simulink model "ModeleringBevegelserSim"  (R2023b)
settings: Solver=FixedStepAuto  StartTime=0.0  StopTime=6  FixedStep=1e-3  RelTol=1e-6
undefined symbols (not defined in the file): areal_front, areal_side, areal_topp, bidrag_gir_front, bidrag_gir_side, Cd_front, Cd_side, Cd_topp, g, masse, r_motor_gir, tetthet_vann, theta_motor_gir, treghetsmoment_gir
libraries: spsFirstOrderFilterLib x4, slpidlib x4
settings Model: Creator=bmm1  LastModifiedBy=bmm1

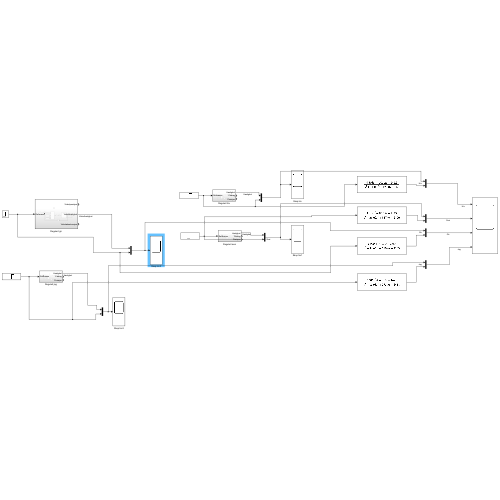
[thumbnail: Simulink's stored preview of the top-level diagram]
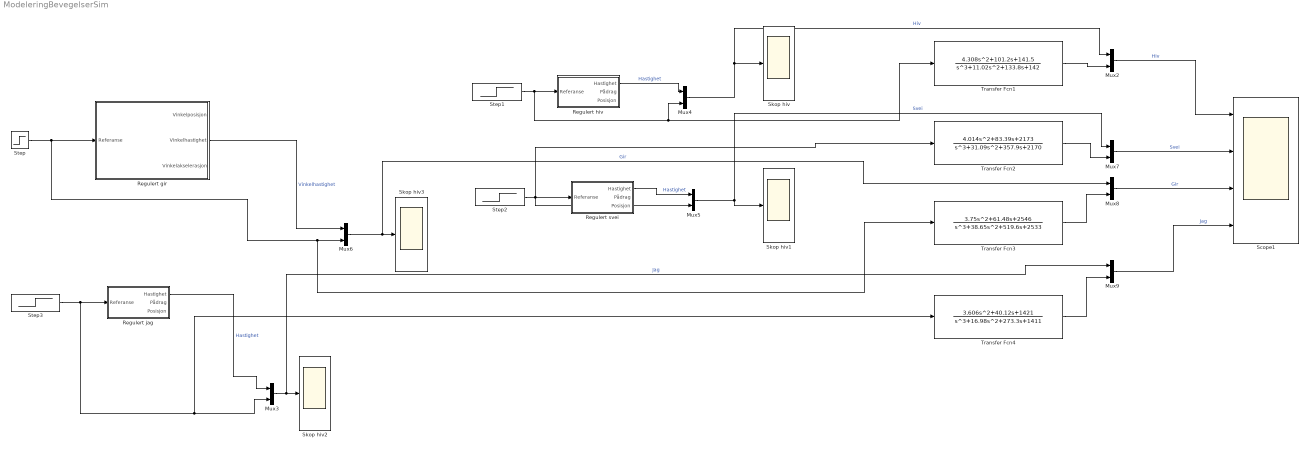
== system ModeleringBevegelserSim ==
  Mux{2..9} (8 alike) : Mux  Inputs=2
  "Regulert gir " : Subsystem
  Regulert hiv : Subsystem
  Regulert jag : Subsystem
  Regulert svei : Subsystem
  Scope1 : Scope  NumInputPorts=4
  Skop hiv{,1..3} (4 alike) : Scope
  Step : Step  SampleTime=0
  Step1 : Step  After=0.6  SampleTime=0
  Step2 : Step  After=0.4  SampleTime=0
  Step3 : Step  After=0.6  SampleTime=0
  Transfer Fcn1 : TransferFcn  Numerator=[4.308 101.2 141.5]  Denominator=[1 11.02 133.8 142]
  Transfer Fcn2 : TransferFcn  Numerator=[4.014 83.39 2173]  Denominator=[1 31.09 357.9 2170]
  Transfer Fcn3 : TransferFcn  Numerator=[3.75 61.48 2546]  Denominator=[1 38.65 519.6 2533]
  Transfer Fcn4 : TransferFcn  Numerator=[3.606 40.12 1421]  Denominator=[1 16.98 273.3 1411]
  wires:
  "Regulert gir "/2(Vinkelhastighet) -> Mux6/1  "Vinkelhastighet"
  Step/1 -> Transfer Fcn3/1, Mux6/2, "Regulert gir "/1(Referanse)
  Step1/1 -> Transfer Fcn1/1, Mux4/2, Regulert hiv/1(Referanse)
  Regulert hiv/1(Hastighet) -> Mux4/1  "Hastighet"
  Step2/1 -> Regulert svei/1(Referanse), Transfer Fcn2/1, Mux5/2
  Step3/1 -> Transfer Fcn4/1, Mux3/2, Regulert jag/1(Referanse)
  Regulert jag/1(Hastighet) -> Mux3/1  "Hastighet"
  Regulert svei/1(Hastighet) -> Mux5/1  "Hastighet"
  Mux5/1 -> Mux7/1, Skop hiv1/1  "Svei"
  Mux4/1 -> Mux2/1, Skop hiv/1  "Hiv"
  Mux6/1 -> Mux8/1, Skop hiv3/1  "Gir"
  Mux3/1 -> Mux9/1, Skop hiv2/1  "Jag"
  Mux2/1 -> Scope1/1  "Hiv"
  Mux7/1 -> Scope1/2  "Svei"
  Mux8/1 -> Scope1/3  "Gir"
  Mux9/1 -> Scope1/4  "Jag"
  Transfer Fcn4/1 -> Mux9/2
  Transfer Fcn3/1 -> Mux8/2
  Transfer Fcn2/1 -> Mux7/2
  Transfer Fcn1/1 -> Mux2/2

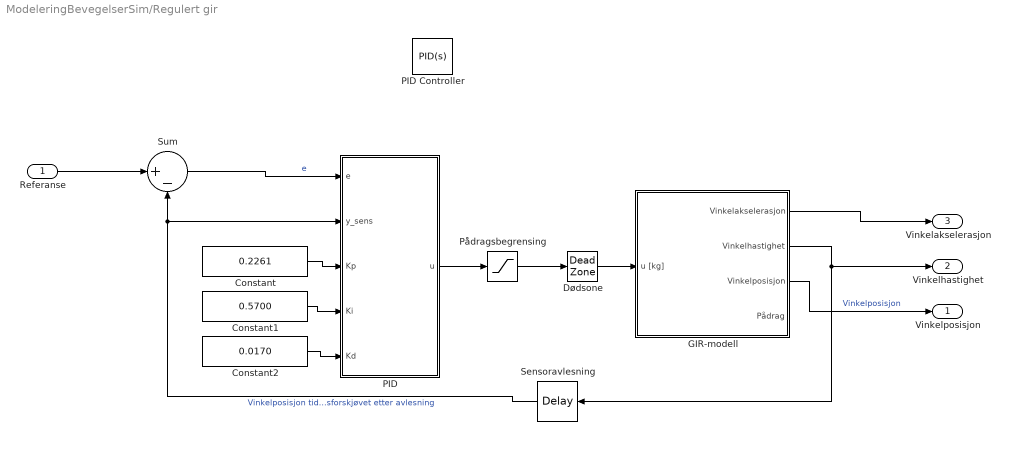
== system ModeleringBevegelserSim/Regulert gir  ==
  Referanse : Inport
  Constant : Constant  Value=0.2261
  Constant1 : Constant  Value=0.5700
  Constant2 : Constant  Value=0.0170
  Dødsone : DeadZone  LowerValue=-0.05  UpperValue=0.05
  GIR-modell : Subsystem
  PID : Subsystem
  PID Controller : slpidlib/PID Controller  Controller=PID  Form=Parallel  TimeDomain=Continuous-time  UseExternalTs=off  SampleTime=-1  IntegratorMethod=Forward Euler  FilterMethod=Forward Euler  ControllerParametersSource=internal  P=0.226088828856197  I=0.0700038160387747  UseKiTs=off  D=0.0170252775761743  N=18.1556932563788  UseFilter=on  TunerSelectOption=Transfer Function Based (PID Tuner App)  InitialConditionSource=internal  InitialConditionForIntegrator=0  InitialConditionForFilter=0  DifferentiatorICPrevScaledInput=0  ExternalReset=none  TrackingMode=off  Kt=1  LimitOutput=off  SatLimitsSource=internal  UpperSaturationLimit=inf  LowerSaturationLimit=-inf  LinearizeAsGain=on  AntiWindupMode=none  Kb=1  LimitIntegrator=off  UpperIntegratorSaturationLimit=inf  LowerIntegratorSaturationLimit=-inf  POutMin=[]  POutMax=[]  IOutMin=[]  IOutMax=[]  DOutMin=[]  DOutMax=[]  NOutMin=[]  NOutMax=[]  SumOutMin=[]  SumOutMax=[]  SaturationOutMin=[]  SaturationOutMax=[]  PParamMin=[]  PParamMax=[]  IParamMin=[]  IParamMax=[]  DParamMin=[]  DParamMax=[]  NParamMin=[]  NParamMax=[]  KbParamMin=[]  KbParamMax=[]  KtParamMin=[]  KtParamMax=[]  KbOutMin=[]  KbOutMax=[]  KtOutMin=[]  KtOutMax=[]  IntegratorOutMin=[]  IntegratorOutMax=[]  FilterOutMin=[]  FilterOutMax=[]  SumI1OutMin=[]  SumI1OutMax=[]  SumI2OutMin=[]  SumI2OutMax=[]  SumI3OutMin=[]  SumI3OutMax=[]  SumI4OutMin=[]  SumI4OutMax=[]  SumDOutMin=[]  SumDOutMax=[]  DifferentiatorOutMin=[]  DifferentiatorOutMax=[]  FilterDiffOutCoefMin=[]  FilterDiffOutCoefMax=[]  ReciprocalOutMin=[]  ReciprocalOutMax=[]  SumDenOutMin=[]  SumDenOutMax=[]  SumNumOutMin=[]  SumNumOutMax=[]  DivideOutMin=[]  DivideOutMax=[]  UdiffTsProdOutMin=[]  UdiffTsProdOutMax=[]  NTsProdOutMin=[]  NTsProdOutMax=[]  UintegralTsProdOutMin=[]  UintegralTsProdOutMax=[]  UngainTsProdOutMin=[]  UngainTsProdOutMax=[]  ClampingZeroOutDataTypeStr=Inherit: Inherit via back propagation  ClampingZeroOutMin=[]  ClampingZeroOutMax=[]  FilterDenConstantOutDataTypeStr=Inherit: Inherit via back propagation  FilterDenConstantOutMin=[]  FilterDenConstantOutMax=[]  PCopyOutDataTypeStr=Inherit: Inherit via back propagation  PCopyOutMin=[]  PCopyOutMax=[]  NCopyOutDataTypeStr=Inherit: Inherit via back propagation  NCopyOutMin=[]  NCopyOutMax=[]  IntegratorContinuousStateAttributes=''  IntegratorStateMustResolveToSignalObject=off  IntegratorRTWStateStorageClass=Auto  FilterContinuousStateAttributes=''  FilterStateMustResolveToSignalObject=off  FilterRTWStateStorageClass=Auto  ParallelPVariant=InternalParameters  IdealPVariant=Disabled  IVariant=InternalParameters  DVariant=InternalParameters  IntegratorVariant=Continuous  SatVariant=Disabled  AWVariant=Passthrough  PCopyVariant=Disabled  TRVariant=Disabled  FdbkBlocksVariant=Forward  IdealPFdbkVariant=Disabled  SatFdbkVariant=Disabled  DerivativeFilterVariant=ContFilter  NVariant=InternalParameters  NCopyVariant=Disabled  FilterICVariant=InternalICsFilter  IntegratorICVariant=InternalICs  ExternalResetVariant=Disabled  TRSumVariant=Passthrough  SumFdbkVariant=Disabled  SumVariant=Sum_PID  TsampFilterVariant=InternalTs  TsampNgainVariant=Passthrough  TsampIntegralVariant=Disabled_SignalSpec  ExternalSaturationOutDataTypeStr=Inherit: Same as second input
  Pådragsbegrensing : Saturate  UpperLimit=2.7  LowerLimit=-2.7
  Sensoravlesning : TransportDelay  DelayTime=0.2
  Sum : Sum  Inputs=|+-
  Vinkelposisjon : Outport
  Vinkelhastighet : Outport  Port=2
  Vinkelakselerasjon : Outport  Port=3
  wires:
  Constant1/1 -> PID/4(Ki)
  Constant/1 -> PID/3(Kp)
  Constant2/1 -> PID/5(Kd)
  Sum/1 -> PID/1(e)  "e"
  GIR-modell/3(Vinkelposisjon) -> Vinkelposisjon/1  "Vinkelposisjon"
  GIR-modell/2(" Vinkelhastighet") -> Vinkelhastighet/1, Sensoravlesning/1
  GIR-modell/1(" Vinkelakselerasjon") -> Vinkelakselerasjon/1
  Referanse/1 -> Sum/1
  Sensoravlesning/1 -> Sum/2, PID/2(y_sens)  "Vinkelposisjon tidsforskjøvet etter avlesning"
  Pådragsbegrensing/1 -> Dødsone/1
  Dødsone/1 -> GIR-modell/1(u [kg])
  PID/1(u) -> Pådragsbegrensing/1

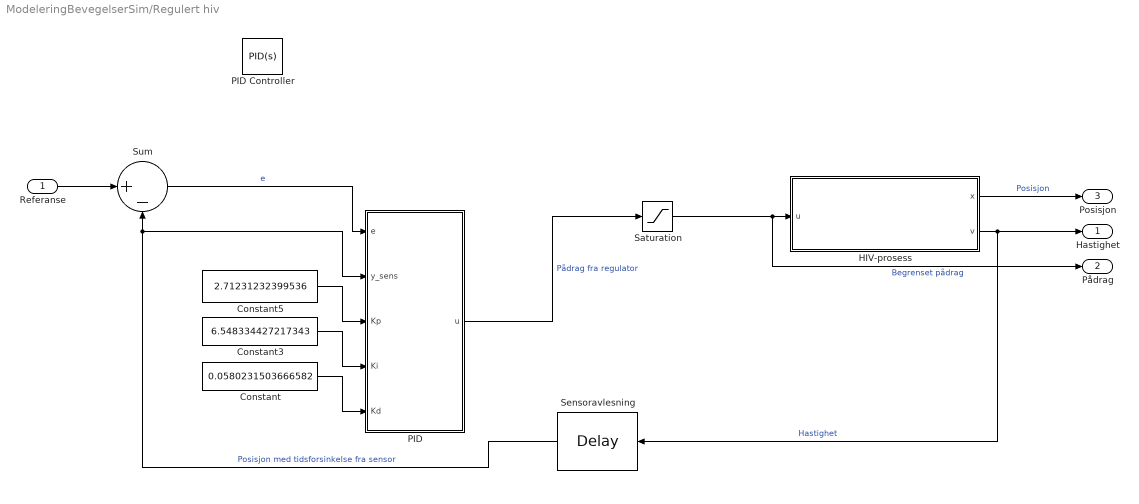
== system ModeleringBevegelserSim/Regulert hiv ==
  Referanse : Inport
  Constant : Constant  Value=0.0580231503666582
  Constant3 : Constant  Value=6.548334427217343
  Constant5 : Constant  Value=2.71231232399536
  HIV-prosess : Subsystem
      settings: AttributesFormatString=Hiv-modell
  PID : Subsystem
  PID Controller : slpidlib/PID Controller  Controller=PID  Form=Parallel  TimeDomain=Continuous-time  UseExternalTs=off  SampleTime=-1  IntegratorMethod=Forward Euler  FilterMethod=Forward Euler  ControllerParametersSource=internal  P=1.71231232399536  I=0.548334427217343  UseKiTs=off  D=0.0580231503666582  N=35.6308273811932  UseFilter=on  TunerSelectOption=Transfer Function Based (PID Tuner App)  InitialConditionSource=internal  InitialConditionForIntegrator=0  InitialConditionForFilter=0  DifferentiatorICPrevScaledInput=0  ExternalReset=none  TrackingMode=off  Kt=1  LimitOutput=off  SatLimitsSource=internal  UpperSaturationLimit=inf  LowerSaturationLimit=-inf  LinearizeAsGain=on  AntiWindupMode=none  Kb=1  LimitIntegrator=off  UpperIntegratorSaturationLimit=inf  LowerIntegratorSaturationLimit=-inf  POutMin=[]  POutMax=[]  IOutMin=[]  IOutMax=[]  DOutMin=[]  DOutMax=[]  NOutMin=[]  NOutMax=[]  SumOutMin=[]  SumOutMax=[]  SaturationOutMin=[]  SaturationOutMax=[]  PParamMin=[]  PParamMax=[]  IParamMin=[]  IParamMax=[]  DParamMin=[]  DParamMax=[]  NParamMin=[]  NParamMax=[]  KbParamMin=[]  KbParamMax=[]  KtParamMin=[]  KtParamMax=[]  KbOutMin=[]  KbOutMax=[]  KtOutMin=[]  KtOutMax=[]  IntegratorOutMin=[]  IntegratorOutMax=[]  FilterOutMin=[]  FilterOutMax=[]  SumI1OutMin=[]  SumI1OutMax=[]  SumI2OutMin=[]  SumI2OutMax=[]  SumI3OutMin=[]  SumI3OutMax=[]  SumI4OutMin=[]  SumI4OutMax=[]  SumDOutMin=[]  SumDOutMax=[]  DifferentiatorOutMin=[]  DifferentiatorOutMax=[]  FilterDiffOutCoefMin=[]  FilterDiffOutCoefMax=[]  ReciprocalOutMin=[]  ReciprocalOutMax=[]  SumDenOutMin=[]  SumDenOutMax=[]  SumNumOutMin=[]  SumNumOutMax=[]  DivideOutMin=[]  DivideOutMax=[]  UdiffTsProdOutMin=[]  UdiffTsProdOutMax=[]  NTsProdOutMin=[]  NTsProdOutMax=[]  UintegralTsProdOutMin=[]  UintegralTsProdOutMax=[]  UngainTsProdOutMin=[]  UngainTsProdOutMax=[]  ClampingZeroOutDataTypeStr=Inherit: Inherit via back propagation  ClampingZeroOutMin=[]  ClampingZeroOutMax=[]  FilterDenConstantOutDataTypeStr=Inherit: Inherit via back propagation  FilterDenConstantOutMin=[]  FilterDenConstantOutMax=[]  PCopyOutDataTypeStr=Inherit: Inherit via back propagation  PCopyOutMin=[]  PCopyOutMax=[]  NCopyOutDataTypeStr=Inherit: Inherit via back propagation  NCopyOutMin=[]  NCopyOutMax=[]  IntegratorContinuousStateAttributes=''  IntegratorStateMustResolveToSignalObject=off  IntegratorRTWStateStorageClass=Auto  FilterContinuousStateAttributes=''  FilterStateMustResolveToSignalObject=off  FilterRTWStateStorageClass=Auto  ParallelPVariant=InternalParameters  IdealPVariant=Disabled  IVariant=InternalParameters  DVariant=InternalParameters  IntegratorVariant=Continuous  SatVariant=Disabled  AWVariant=Passthrough  PCopyVariant=Disabled  TRVariant=Disabled  FdbkBlocksVariant=Forward  IdealPFdbkVariant=Disabled  SatFdbkVariant=Disabled  DerivativeFilterVariant=ContFilter  NVariant=InternalParameters  NCopyVariant=Disabled  FilterICVariant=InternalICsFilter  IntegratorICVariant=InternalICs  ExternalResetVariant=Disabled  TRSumVariant=Passthrough  SumFdbkVariant=Disabled  SumVariant=Sum_PID  TsampFilterVariant=InternalTs  TsampNgainVariant=Passthrough  TsampIntegralVariant=Disabled_SignalSpec  ExternalSaturationOutDataTypeStr=Inherit: Same as second input
  Saturation : Saturate  UpperLimit=2.7  LowerLimit=-2.7
  Sensoravlesning : TransportDelay  DelayTime=0.2
  Sum : Sum  Inputs=|+-
  Hastighet : Outport
  Pådrag : Outport  Port=2
  Posisjon : Outport  Port=3
  wires:
  PID/1(u) -> Saturation/1  "Pådrag fra regulator"
  Sum/1 -> PID/1(e)  "e"
  Constant/1 -> PID/5(Kd)
  Sensoravlesning/1 -> Sum/2, PID/2(y_sens)  "Posisjon med tidsforsinkelse fra sensor"
  HIV-prosess/1(x) -> Posisjon/1  "Posisjon"
  HIV-prosess/2(v) -> Sensoravlesning/1, Hastighet/1  "Hastighet"
  Referanse/1 -> Sum/1
  Saturation/1 -> HIV-prosess/1(u), Pådrag/1  "Begrenset pådrag"
  Constant3/1 -> PID/4(Ki)
  Constant5/1 -> PID/3(Kp)

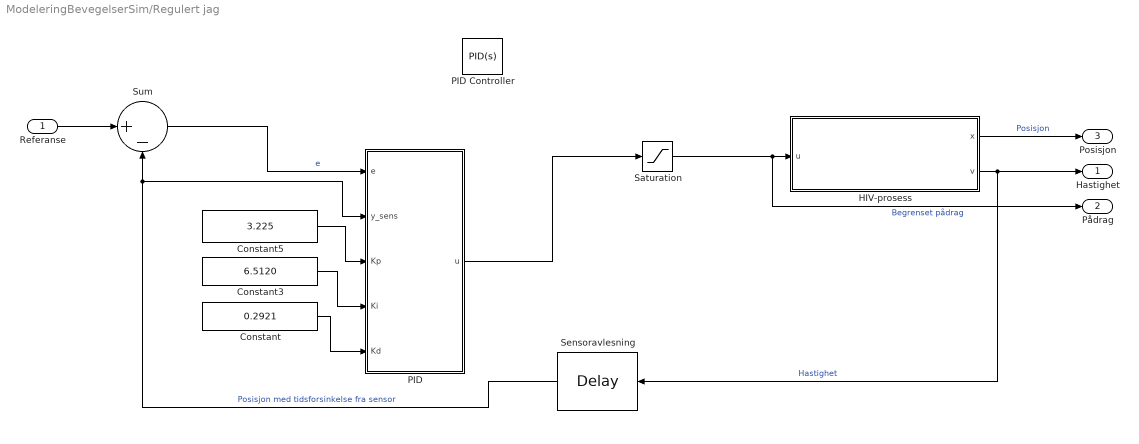
== system ModeleringBevegelserSim/Regulert jag ==
  Referanse : Inport
  Constant : Constant  Value=0.2921
  Constant3 : Constant  Value=6.5120
  Constant5 : Constant  Value=3.225
  HIV-prosess : Subsystem
      settings: AttributesFormatString=Jag modell
  PID : Subsystem
  PID Controller : slpidlib/PID Controller  Controller=PID  Form=Parallel  TimeDomain=Continuous-time  UseExternalTs=off  SampleTime=-1  IntegratorMethod=Forward Euler  FilterMethod=Forward Euler  ControllerParametersSource=internal  P=3.22259477110725  I=1.01234778879115  UseKiTs=off  D=0.292163696521639  N=18.5257141787235  UseFilter=on  TunerSelectOption=Transfer Function Based (PID Tuner App)  InitialConditionSource=internal  InitialConditionForIntegrator=0  InitialConditionForFilter=0  DifferentiatorICPrevScaledInput=0  ExternalReset=none  TrackingMode=off  Kt=1  LimitOutput=off  SatLimitsSource=internal  UpperSaturationLimit=inf  LowerSaturationLimit=-inf  LinearizeAsGain=on  AntiWindupMode=none  Kb=1  LimitIntegrator=off  UpperIntegratorSaturationLimit=inf  LowerIntegratorSaturationLimit=-inf  POutMin=[]  POutMax=[]  IOutMin=[]  IOutMax=[]  DOutMin=[]  DOutMax=[]  NOutMin=[]  NOutMax=[]  SumOutMin=[]  SumOutMax=[]  SaturationOutMin=[]  SaturationOutMax=[]  PParamMin=[]  PParamMax=[]  IParamMin=[]  IParamMax=[]  DParamMin=[]  DParamMax=[]  NParamMin=[]  NParamMax=[]  KbParamMin=[]  KbParamMax=[]  KtParamMin=[]  KtParamMax=[]  KbOutMin=[]  KbOutMax=[]  KtOutMin=[]  KtOutMax=[]  IntegratorOutMin=[]  IntegratorOutMax=[]  FilterOutMin=[]  FilterOutMax=[]  SumI1OutMin=[]  SumI1OutMax=[]  SumI2OutMin=[]  SumI2OutMax=[]  SumI3OutMin=[]  SumI3OutMax=[]  SumI4OutMin=[]  SumI4OutMax=[]  SumDOutMin=[]  SumDOutMax=[]  DifferentiatorOutMin=[]  DifferentiatorOutMax=[]  FilterDiffOutCoefMin=[]  FilterDiffOutCoefMax=[]  ReciprocalOutMin=[]  ReciprocalOutMax=[]  SumDenOutMin=[]  SumDenOutMax=[]  SumNumOutMin=[]  SumNumOutMax=[]  DivideOutMin=[]  DivideOutMax=[]  UdiffTsProdOutMin=[]  UdiffTsProdOutMax=[]  NTsProdOutMin=[]  NTsProdOutMax=[]  UintegralTsProdOutMin=[]  UintegralTsProdOutMax=[]  UngainTsProdOutMin=[]  UngainTsProdOutMax=[]  ClampingZeroOutDataTypeStr=Inherit: Inherit via back propagation  ClampingZeroOutMin=[]  ClampingZeroOutMax=[]  FilterDenConstantOutDataTypeStr=Inherit: Inherit via back propagation  FilterDenConstantOutMin=[]  FilterDenConstantOutMax=[]  PCopyOutDataTypeStr=Inherit: Inherit via back propagation  PCopyOutMin=[]  PCopyOutMax=[]  NCopyOutDataTypeStr=Inherit: Inherit via back propagation  NCopyOutMin=[]  NCopyOutMax=[]  IntegratorContinuousStateAttributes=''  IntegratorStateMustResolveToSignalObject=off  IntegratorRTWStateStorageClass=Auto  FilterContinuousStateAttributes=''  FilterStateMustResolveToSignalObject=off  FilterRTWStateStorageClass=Auto  ParallelPVariant=InternalParameters  IdealPVariant=Disabled  IVariant=InternalParameters  DVariant=InternalParameters  IntegratorVariant=Continuous  SatVariant=Disabled  AWVariant=Passthrough  PCopyVariant=Disabled  TRVariant=Disabled  FdbkBlocksVariant=Forward  IdealPFdbkVariant=Disabled  SatFdbkVariant=Disabled  DerivativeFilterVariant=ContFilter  NVariant=InternalParameters  NCopyVariant=Disabled  FilterICVariant=InternalICsFilter  IntegratorICVariant=InternalICs  ExternalResetVariant=Disabled  TRSumVariant=Passthrough  SumFdbkVariant=Disabled  SumVariant=Sum_PID  TsampFilterVariant=InternalTs  TsampNgainVariant=Passthrough  TsampIntegralVariant=Disabled_SignalSpec  ExternalSaturationOutDataTypeStr=Inherit: Same as second input
  Saturation : Saturate  UpperLimit=2.7  LowerLimit=-2.7
  Sensoravlesning : TransportDelay  DelayTime=0.2
  Sum : Sum  Inputs=|+-
  Hastighet : Outport
  Pådrag : Outport  Port=2
  Posisjon : Outport  Port=3
  wires:
  PID/1(u) -> Saturation/1
  Sum/1 -> PID/1(e)  "e"
  Constant/1 -> PID/5(Kd)
  Sensoravlesning/1 -> Sum/2, PID/2(y_sens)  "Posisjon med tidsforsinkelse fra sensor"
  HIV-prosess/1(x) -> Posisjon/1  "Posisjon"
  HIV-prosess/2(v) -> Sensoravlesning/1, Hastighet/1  "Hastighet"
  Referanse/1 -> Sum/1
  Saturation/1 -> HIV-prosess/1(u), Pådrag/1  "Begrenset pådrag"
  Constant3/1 -> PID/4(Ki)
  Constant5/1 -> PID/3(Kp)

== system ModeleringBevegelserSim/Regulert svei ==
  Referanse : Inport
  Constant : Constant  Value=0.1160
  Constant3 : Constant  Value=10.0966
  Constant5 : Constant  Value=3.4246
  PID : Subsystem
  PID Controller : slpidlib/PID Controller  Controller=PID  Form=Parallel  TimeDomain=Continuous-time  UseExternalTs=off  SampleTime=-1  IntegratorMethod=Forward Euler  FilterMethod=Forward Euler  ControllerParametersSource=internal  P=3.42462464799072  I=1.09666885443469  UseKiTs=off  D=0.116046300733316  N=35.6308273811932  UseFilter=on  TunerSelectOption=Transfer Function Based (PID Tuner App)  InitialConditionSource=internal  InitialConditionForIntegrator=0  InitialConditionForFilter=0  DifferentiatorICPrevScaledInput=0  ExternalReset=none  TrackingMode=off  Kt=1  LimitOutput=off  SatLimitsSource=internal  UpperSaturationLimit=inf  LowerSaturationLimit=-inf  LinearizeAsGain=on  AntiWindupMode=none  Kb=1  LimitIntegrator=off  UpperIntegratorSaturationLimit=inf  LowerIntegratorSaturationLimit=-inf  POutMin=[]  POutMax=[]  IOutMin=[]  IOutMax=[]  DOutMin=[]  DOutMax=[]  NOutMin=[]  NOutMax=[]  SumOutMin=[]  SumOutMax=[]  SaturationOutMin=[]  SaturationOutMax=[]  PParamMin=[]  PParamMax=[]  IParamMin=[]  IParamMax=[]  DParamMin=[]  DParamMax=[]  NParamMin=[]  NParamMax=[]  KbParamMin=[]  KbParamMax=[]  KtParamMin=[]  KtParamMax=[]  KbOutMin=[]  KbOutMax=[]  KtOutMin=[]  KtOutMax=[]  IntegratorOutMin=[]  IntegratorOutMax=[]  FilterOutMin=[]  FilterOutMax=[]  SumI1OutMin=[]  SumI1OutMax=[]  SumI2OutMin=[]  SumI2OutMax=[]  SumI3OutMin=[]  SumI3OutMax=[]  SumI4OutMin=[]  SumI4OutMax=[]  SumDOutMin=[]  SumDOutMax=[]  DifferentiatorOutMin=[]  DifferentiatorOutMax=[]  FilterDiffOutCoefMin=[]  FilterDiffOutCoefMax=[]  ReciprocalOutMin=[]  ReciprocalOutMax=[]  SumDenOutMin=[]  SumDenOutMax=[]  SumNumOutMin=[]  SumNumOutMax=[]  DivideOutMin=[]  DivideOutMax=[]  UdiffTsProdOutMin=[]  UdiffTsProdOutMax=[]  NTsProdOutMin=[]  NTsProdOutMax=[]  UintegralTsProdOutMin=[]  UintegralTsProdOutMax=[]  UngainTsProdOutMin=[]  UngainTsProdOutMax=[]  ClampingZeroOutDataTypeStr=Inherit: Inherit via back propagation  ClampingZeroOutMin=[]  ClampingZeroOutMax=[]  FilterDenConstantOutDataTypeStr=Inherit: Inherit via back propagation  FilterDenConstantOutMin=[]  FilterDenConstantOutMax=[]  PCopyOutDataTypeStr=Inherit: Inherit via back propagation  PCopyOutMin=[]  PCopyOutMax=[]  NCopyOutDataTypeStr=Inherit: Inherit via back propagation  NCopyOutMin=[]  NCopyOutMax=[]  IntegratorContinuousStateAttributes=''  IntegratorStateMustResolveToSignalObject=off  IntegratorRTWStateStorageClass=Auto  FilterContinuousStateAttributes=''  FilterStateMustResolveToSignalObject=off  FilterRTWStateStorageClass=Auto  ParallelPVariant=InternalParameters  IdealPVariant=Disabled  IVariant=InternalParameters  DVariant=InternalParameters  IntegratorVariant=Continuous  SatVariant=Disabled  AWVariant=Passthrough  PCopyVariant=Disabled  TRVariant=Disabled  FdbkBlocksVariant=Forward  IdealPFdbkVariant=Disabled  SatFdbkVariant=Disabled  DerivativeFilterVariant=ContFilter  NVariant=InternalParameters  NCopyVariant=Disabled  FilterICVariant=InternalICsFilter  IntegratorICVariant=InternalICs  ExternalResetVariant=Disabled  TRSumVariant=Passthrough  SumFdbkVariant=Disabled  SumVariant=Sum_PID  TsampFilterVariant=InternalTs  TsampNgainVariant=Passthrough  TsampIntegralVariant=Disabled_SignalSpec  ExternalSaturationOutDataTypeStr=Inherit: Same as second input
  Saturation : Saturate  UpperLimit=2.7  LowerLimit=-2.7
  Sensoravlesning : TransportDelay  DelayTime=0.2
  Sum : Sum  Inputs=|+-
  svai-prosess : Subsystem
      settings: AttributesFormatString=Svei modell
  Hastighet : Outport
  Pådrag : Outport  Port=2
  Posisjon : Outport  Port=3
  wires:
  PID/1(u) -> Saturation/1
  Sum/1 -> PID/1(e)  "e"
  Constant/1 -> PID/5(Kd)
  Sensoravlesning/1 -> Sum/2, PID/2(y_sens)  "Posisjon med tidsforsinkelse fra sensor"
  svai-prosess/1(x) -> Posisjon/1  "Posisjon"
  svai-prosess/2(v) -> Sensoravlesning/1, Hastighet/1  "Hastighet"
  Referanse/1 -> Sum/1
  Saturation/1 -> svai-prosess/1(u), Pådrag/1  "Begrenset pådrag"
  Constant3/1 -> PID/4(Ki)
  Constant5/1 -> PID/3(Kp)

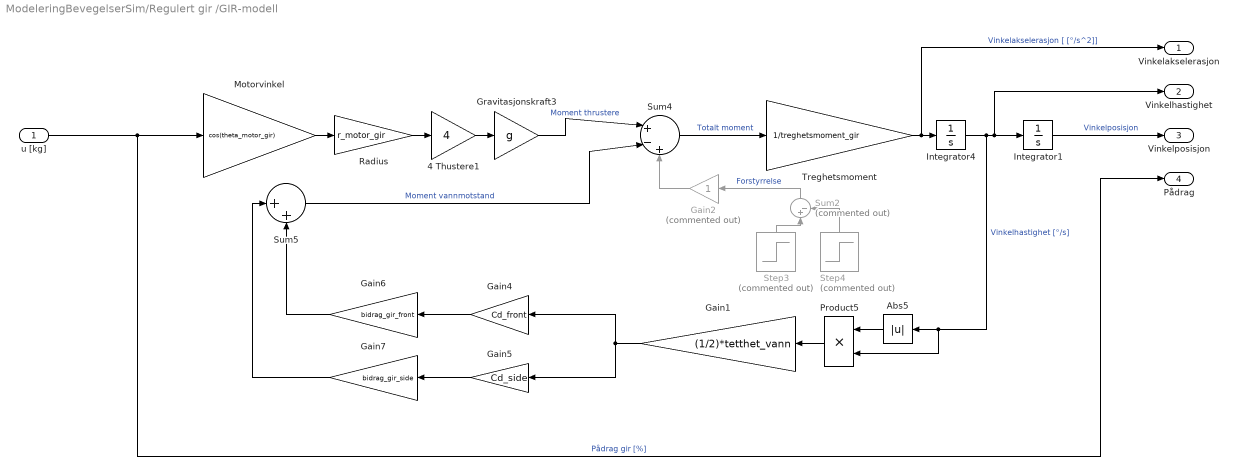
== system ModeleringBevegelserSim/Regulert gir /GIR-modell ==
  u [kg] : Inport
  4 Thustere1 : Gain  Gain=4
  Abs5 : Abs  SaturateOnIntegerOverflow=off
  Gain1 : Gain  Gain=(1/2)*tetthet_vann
  Gain2 : Gain  Commented=on
  Gain4 : Gain  Gain=Cd_front
  Gain5 : Gain  Gain=Cd_side
  Gain6 : Gain  Gain=bidrag_gir_front
  Gain7 : Gain  Gain=bidrag_gir_side
  Gravitasjonskraft3 : Gain  Gain=g
  Integrator1 : Integrator
  Integrator4 : Integrator
  Motorvinkel : Gain  Gain=cos(theta_motor_gir)
  Product5 : Product
  Radius : Gain  Gain=r_motor_gir
  Step3 : Step  Commented=on  Time=10  After=0.5  SampleTime=0
  Step4 : Step  Commented=on  Time=25  After=0.5  SampleTime=0
  Sum2 : Sum  Commented=on  Inputs=|+-
  Sum4 : Sum  Inputs=|+-+
  Sum5 : Sum  Inputs=|++
  Treghetsmoment : Gain  Gain=1/treghetsmoment_gir
  " Vinkelakselerasjon" : Outport
  " Vinkelhastighet" : Outport  Port=2
  Vinkelposisjon : Outport  Port=3
  " Pådrag" : Outport  Port=4
  wires:
  Gain4/1 -> Gain6/1
  Radius/1 -> 4 Thustere1/1
  Sum4/1 -> Treghetsmoment/1  "Totalt moment"
  Abs5/1 -> Product5/1
  Product5/1 -> Gain1/1
  Sum5/1 -> Sum4/2  "Moment vannmotstand"
  Gain6/1 -> Sum5/2
  Gain7/1 -> Sum5/1
  Gravitasjonskraft3/1 -> Sum4/1  "Moment thrustere"
  Gain1/1 -> Gain5/1, Gain4/1
  Gain5/1 -> Gain7/1
  u [kg]/1 -> " Pådrag"/1, Motorvinkel/1  "Pådrag gir [%]"
  Motorvinkel/1 -> Radius/1
  Integrator4/1 -> " Vinkelhastighet"/1, Integrator1/1, Abs5/1, Product5/2  "Vinkelhastighet [°/s]"
  4 Thustere1/1 -> Gravitasjonskraft3/1
  Treghetsmoment/1 -> " Vinkelakselerasjon"/1, Integrator4/1  "Vinkelakselerasjon [ [°/s^2]]"
  Sum2/1 -> Gain2/1  "Forstyrrelse"
  Step4/1 -> Sum2/2
  Step3/1 -> Sum2/1
  Integrator1/1 -> Vinkelposisjon/1  "Vinkelposisjon"
  Gain2/1 -> Sum4/3

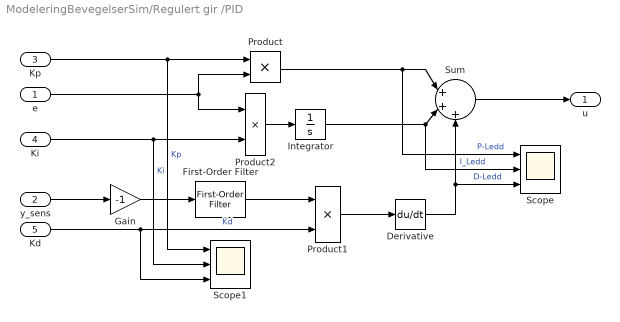
== system ModeleringBevegelserSim/Regulert gir /PID ==
  e : Inport
  y_sens : Inport  Port=2
  Kp : Inport  Port=3
  Ki : Inport  Port=4
  Kd : Inport  Port=5
  Derivative : Derivative
  First-Order Filter : spsFirstOrderFilterLib/First-Order Filter  FilterType=Lowpass  Tc=(0.11/0.14)*0.05  Ts=0  Initialize=on  Vac_Init=[0, 0, 60]  Vdc_Init=0  PlotResponse=off  FreqRange="[0,  200,  1]"
  Gain : Gain  Gain=-1
  Integrator : Integrator  LimitOutput=on
  Product : Product
  Product1 : Product
  Product2 : Product
  Scope : Scope  NumInputPorts=3
  Scope1 : Scope  NumInputPorts=3
  Sum : Sum  Inputs=|+++
  u : Outport
  wires:
  e/1 -> Product2/1, Product/2
  Sum/1 -> u/1
  y_sens/1 -> Gain/1
  Kd/1 -> Scope1/3, Product1/2  "Kd"
  Ki/1 -> Scope1/2, Product2/2  "Ki"
  Product2/1 -> Integrator/1
  Product1/1 -> Derivative/1
  Derivative/1 -> Sum/3, Scope/3  "D-Ledd"
  Product/1 -> Scope/1, Sum/1  "P-Ledd"
  Integrator/1 -> Sum/2, Scope/2  "I_Ledd"
  Kp/1 -> Scope1/1, Product/1  "Kp"
  Gain/1 -> First-Order Filter/1
  First-Order Filter/1 -> Product1/1

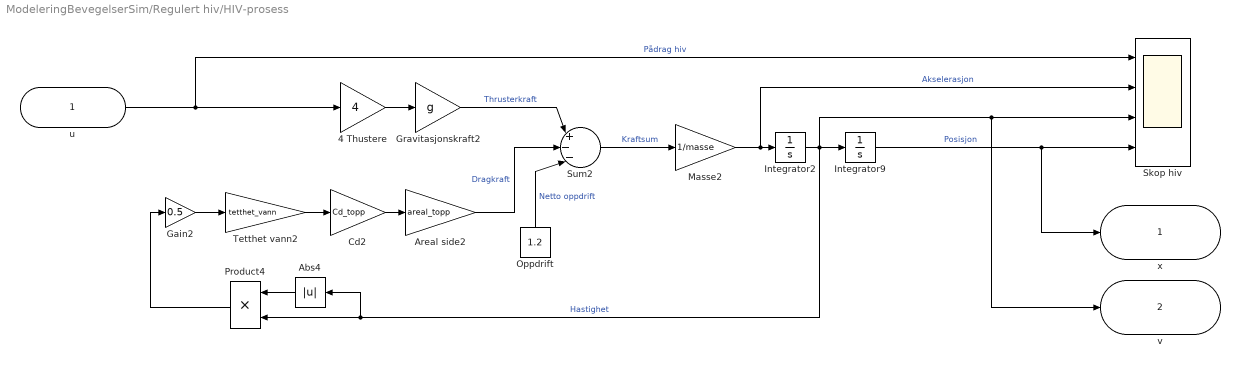
== system ModeleringBevegelserSim/Regulert hiv/HIV-prosess ==
  u : Inport
  4 Thustere : Gain  Gain=4
  Abs4 : Abs  SaturateOnIntegerOverflow=off
  Areal side2 : Gain  Gain=areal_topp
  Cd2 : Gain  Gain=Cd_topp
  Gain2 : Gain  Gain=0.5
  Gravitasjonskraft2 : Gain  Gain=g
  Integrator2 : Integrator
  Integrator9 : Integrator
  Masse2 : Gain  Gain=1/masse
  Oppdrift : Constant  Value=1.2
  Product4 : Product
  Skop hiv : Scope  NumInputPorts=4
  Sum2 : Sum  Inputs=|+--|
  Tetthet vann2 : Gain  Gain=tetthet_vann
  x : Outport
  v : Outport  Port=2
  wires:
  Abs4/1 -> Product4/1
  4 Thustere/1 -> Gravitasjonskraft2/1
  Cd2/1 -> Areal side2/1
  Tetthet vann2/1 -> Cd2/1
  Sum2/1 -> Masse2/1  "Kraftsum"
  Areal side2/1 -> Sum2/2  "Dragkraft"
  Masse2/1 -> Skop hiv/2, Integrator2/1  "Akselerasjon"
  Gain2/1 -> Tetthet vann2/1
  Gravitasjonskraft2/1 -> Sum2/1  "Thrusterkraft"
  Oppdrift/1 -> Sum2/3  "Netto oppdrift"
  Integrator2/1 -> Abs4/1, Product4/2, Integrator9/1, v/1, Skop hiv/3  "Hastighet"
  Product4/1 -> Gain2/1
  u/1 -> Skop hiv/1, 4 Thustere/1  "Pådrag hiv"
  Integrator9/1 -> x/1, Skop hiv/4  "Posisjon"

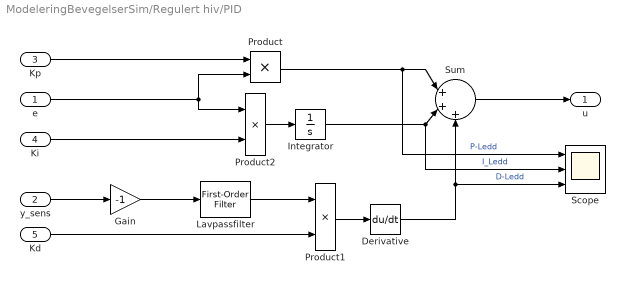
== system ModeleringBevegelserSim/Regulert hiv/PID ==
  e : Inport
  y_sens : Inport  Port=2
  Kp : Inport  Port=3
  Ki : Inport  Port=4
  Kd : Inport  Port=5
  Derivative : Derivative
  Gain : Gain  Gain=-1
  Integrator : Integrator  LimitOutput=on  UpperSaturationLimit=2  LowerSaturationLimit=-0.15
  Lavpassfilter : spsFirstOrderFilterLib/First-Order Filter  FilterType=Lowpass  Tc=(1.27/1.59)*0.05  Ts=0  Initialize=on  Vac_Init=[0, 0, 60]  Vdc_Init=0  PlotResponse=off  FreqRange="[0,  200,  1]"
  Product : Product
  Product1 : Product
  Product2 : Product
  Scope : Scope  NumInputPorts=3
  Sum : Sum  Inputs=|+++
  u : Outport
  wires:
  e/1 -> Product/2, Product2/1
  Sum/1 -> u/1
  y_sens/1 -> Gain/1
  Lavpassfilter/1 -> Product1/1
  Kd/1 -> Product1/2
  Ki/1 -> Product2/2
  Product2/1 -> Integrator/1
  Product1/1 -> Derivative/1
  Derivative/1 -> Sum/3, Scope/3  "D-Ledd"
  Gain/1 -> Lavpassfilter/1
  Product/1 -> Scope/1, Sum/1  "P-Ledd"
  Integrator/1 -> Sum/2, Scope/2  "I_Ledd"
  Kp/1 -> Product/1

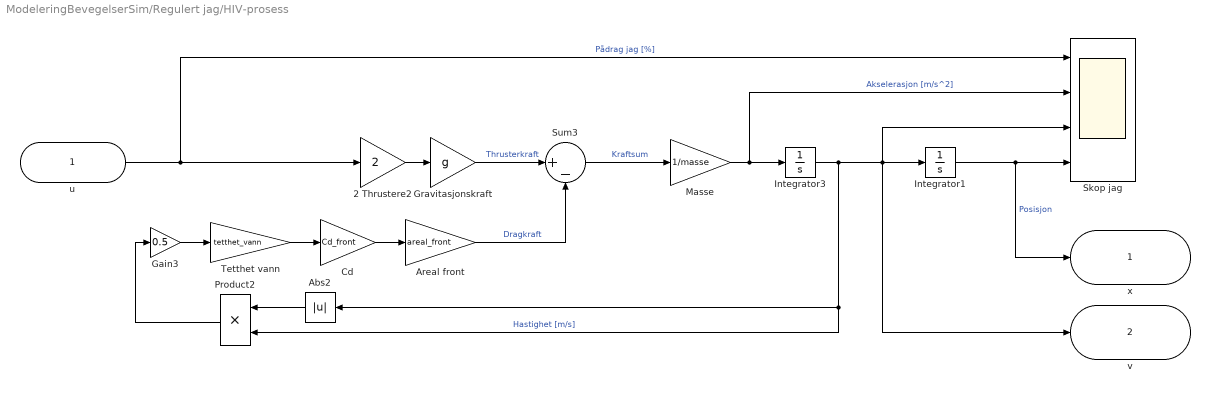
== system ModeleringBevegelserSim/Regulert jag/HIV-prosess ==
  u : Inport
  2 Thrustere2 : Gain  Gain=2
  Abs2 : Abs  SaturateOnIntegerOverflow=off
  Areal front : Gain  Gain=areal_front
  Cd : Gain  Gain=Cd_front
  Gain3 : Gain  Gain=0.5
  Gravitasjonskraft : Gain  Gain=g
  Integrator1 : Integrator
  Integrator3 : Integrator
  Masse : Gain  Gain=1/masse
  Product2 : Product
  Skop jag : Scope  NumInputPorts=4
  Sum3 : Sum  Inputs=|+-
  Tetthet vann : Gain  Gain=tetthet_vann
  x : Outport
  v : Outport  Port=2
  wires:
  Integrator3/1 -> Product2/2, Abs2/1, v/1, Skop jag/3, Integrator1/1  "Hastighet [m/s]"
  Cd/1 -> Areal front/1
  Abs2/1 -> Product2/1
  u/1 -> 2 Thrustere2/1, Skop jag/1  "Pådrag jag [%]"
  Areal front/1 -> Sum3/2  "Dragkraft"
  Tetthet vann/1 -> Cd/1
  Gain3/1 -> Tetthet vann/1
  2 Thrustere2/1 -> Gravitasjonskraft/1
  Gravitasjonskraft/1 -> Sum3/1  "Thrusterkraft"
  Product2/1 -> Gain3/1
  Masse/1 -> Skop jag/2, Integrator3/1  "Akselerasjon [m/s^2]"
  Sum3/1 -> Masse/1  "Kraftsum"
  Integrator1/1 -> x/1, Skop jag/4  "Posisjon"

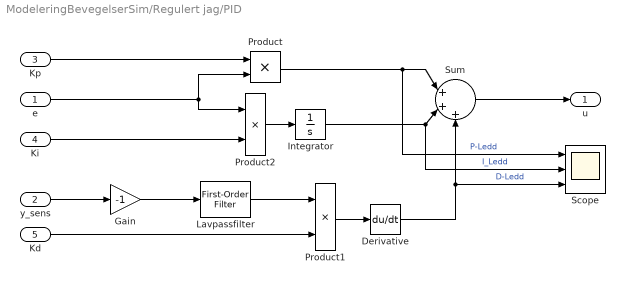
== system ModeleringBevegelserSim/Regulert jag/PID ==
  e : Inport
  y_sens : Inport  Port=2
  Kp : Inport  Port=3
  Ki : Inport  Port=4
  Kd : Inport  Port=5
  Derivative : Derivative
  Gain : Gain  Gain=-1
  Integrator : Integrator  LimitOutput=on  UpperSaturationLimit=2  LowerSaturationLimit=-0.15
  Lavpassfilter : spsFirstOrderFilterLib/First-Order Filter  FilterType=Lowpass  Tc=(1.27/1.59)*0.05  Ts=0  Initialize=on  Vac_Init=[0, 0, 60]  Vdc_Init=0  PlotResponse=off  FreqRange="[0,  200,  1]"
  Product : Product
  Product1 : Product
  Product2 : Product
  Scope : Scope  NumInputPorts=3
  Sum : Sum  Inputs=|+++
  u : Outport
  wires:
  e/1 -> Product/2, Product2/1
  Sum/1 -> u/1
  y_sens/1 -> Gain/1
  Lavpassfilter/1 -> Product1/1
  Kd/1 -> Product1/2
  Ki/1 -> Product2/2
  Product2/1 -> Integrator/1
  Product1/1 -> Derivative/1
  Derivative/1 -> Sum/3, Scope/3  "D-Ledd"
  Gain/1 -> Lavpassfilter/1
  Product/1 -> Scope/1, Sum/1  "P-Ledd"
  Integrator/1 -> Sum/2, Scope/2  "I_Ledd"
  Kp/1 -> Product/1

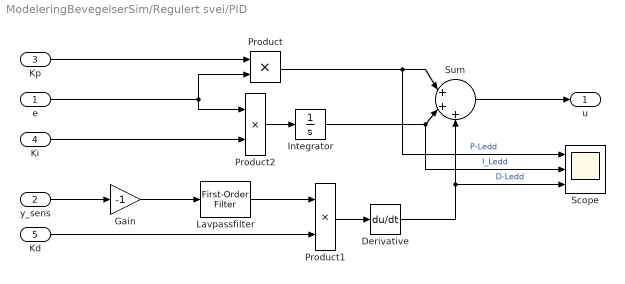
== system ModeleringBevegelserSim/Regulert svei/PID ==
  e : Inport
  y_sens : Inport  Port=2
  Kp : Inport  Port=3
  Ki : Inport  Port=4
  Kd : Inport  Port=5
  Derivative : Derivative
  Gain : Gain  Gain=-1
  Integrator : Integrator  LimitOutput=on  UpperSaturationLimit=2  LowerSaturationLimit=-0.15
  Lavpassfilter : spsFirstOrderFilterLib/First-Order Filter  FilterType=Lowpass  Tc=(1.27/1.59)*0.05  Ts=0  Initialize=on  Vac_Init=[0, 0, 60]  Vdc_Init=0  PlotResponse=off  FreqRange="[0,  200,  1]"
  Product : Product
  Product1 : Product
  Product2 : Product
  Scope : Scope  NumInputPorts=3
  Sum : Sum  Inputs=|+++
  u : Outport
  wires:
  e/1 -> Product/2, Product2/1
  Sum/1 -> u/1
  y_sens/1 -> Gain/1
  Lavpassfilter/1 -> Product1/1
  Kd/1 -> Product1/2
  Ki/1 -> Product2/2
  Product2/1 -> Integrator/1
  Product1/1 -> Derivative/1
  Derivative/1 -> Sum/3, Scope/3  "D-Ledd"
  Gain/1 -> Lavpassfilter/1
  Product/1 -> Scope/1, Sum/1  "P-Ledd"
  Integrator/1 -> Sum/2, Scope/2  "I_Ledd"
  Kp/1 -> Product/1

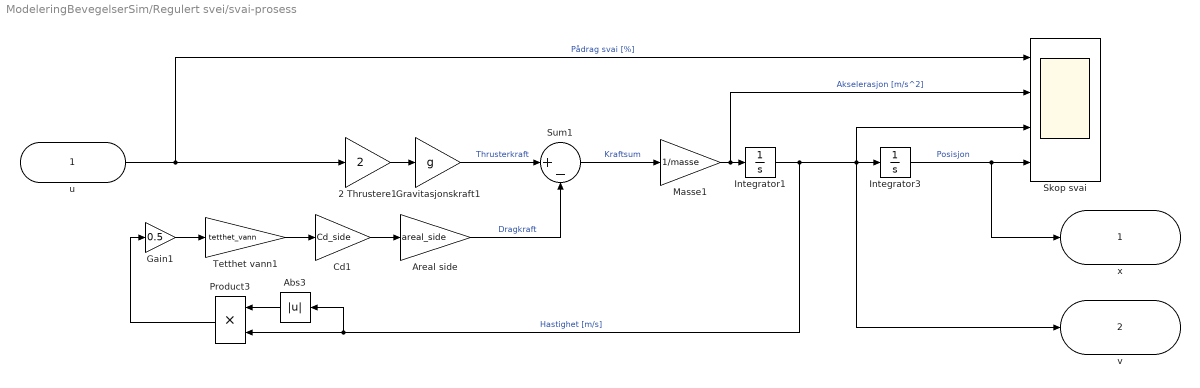
== system ModeleringBevegelserSim/Regulert svei/svai-prosess ==
  u : Inport
  2 Thrustere1 : Gain  Gain=2
  Abs3 : Abs  SaturateOnIntegerOverflow=off
  Areal side : Gain  Gain=areal_side
  Cd1 : Gain  Gain=Cd_side
  Gain1 : Gain  Gain=0.5
  Gravitasjonskraft1 : Gain  Gain=g
  Integrator1 : Integrator
  Integrator3 : Integrator
  Masse1 : Gain  Gain=1/masse
  Product3 : Product
  Skop svai : Scope  NumInputPorts=4
  Sum1 : Sum  Inputs=|+-
  Tetthet vann1 : Gain  Gain=tetthet_vann
  x : Outport
  v : Outport  Port=2
  wires:
  u/1 -> 2 Thrustere1/1, Skop svai/1  "Pådrag svai [%]"
  Gravitasjonskraft1/1 -> Sum1/1  "Thrusterkraft"
  Gain1/1 -> Tetthet vann1/1
  Areal side/1 -> Sum1/2  "Dragkraft"
  Abs3/1 -> Product3/1
  2 Thrustere1/1 -> Gravitasjonskraft1/1
  Cd1/1 -> Areal side/1
  Masse1/1 -> Skop svai/2, Integrator1/1  "Akselerasjon [m/s^2]"
  Product3/1 -> Gain1/1
  Integrator1/1 -> Abs3/1, Product3/2, v/1, Skop svai/3, Integrator3/1  "Hastighet [m/s]"
  Tetthet vann1/1 -> Cd1/1
  Sum1/1 -> Masse1/1  "Kraftsum"
  Integrator3/1 -> x/1, Skop svai/4  "Posisjon"
